simulink subsystem "SensorsInterface"  (R2025b)
settings: Solver=VariableStepAuto  StartTime=0.0  StopTime=10.0  RelTol=1e-3
settings Model: Creator=yvijay  LastModifiedBy=atcushen

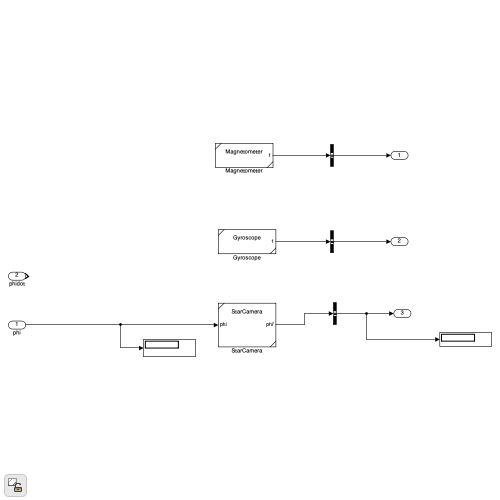
[thumbnail: Simulink's stored preview of the top-level diagram]
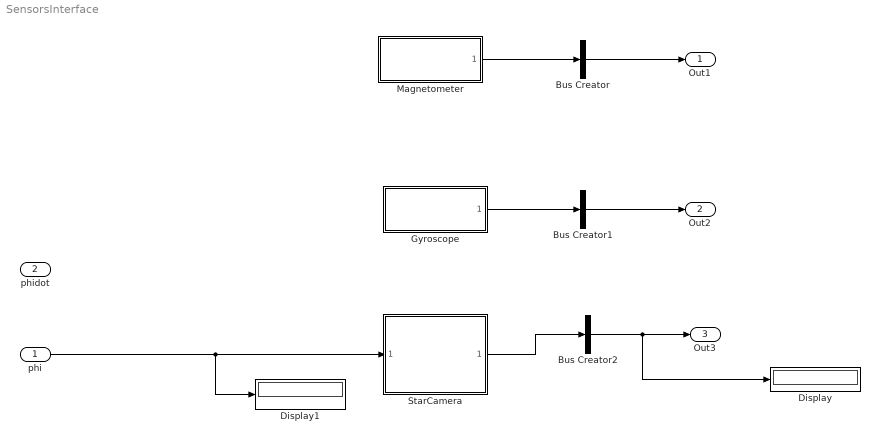
== system SensorsInterface ==
  phi : Inport
  phidot : Inport  Port=2
  Bus Creator : BusCreator  Inputs=1
  Bus Creator1 : BusCreator  Inputs=1
  Bus Creator2 : BusCreator  Inputs=1
  Display : Display
  Display1 : Display
  Gyroscope : Subsystem  ReferencedSubsystem=Gyroscope
  Magnetometer : Subsystem  ReferencedSubsystem=Magnetometer
  StarCamera : Subsystem  ReferencedSubsystem=StarCamera
  Out1 : Outport
  Out2 : Outport  Port=2
  Out3 : Outport  Port=3
  wires:
  Magnetometer/1 -> Bus Creator/1
  Bus Creator/1 -> Out1/1
  Bus Creator1/1 -> Out2/1
  phi/1 -> Display1/1, StarCamera/1
  StarCamera/1 -> Bus Creator2/1
  Gyroscope/1 -> Bus Creator1/1
  Bus Creator2/1 -> Out3/1, Display/1
